simulink model "controller_dev_sg_HIL_noTP"  (R2018b)
settings: configuration reference "Physics" (kept outside this file)
model workspace (MAT data in the model file):
  m = 1000
values from neighbouring files (symbols this model uses):
  bool_activate_Vehicles : value not decoded    [controller_dev_sg.sldd]
  ModObj_ObjList_SendPort = 11004.0    [UDPPortConfig.sldd]
  ModSens_GpsSenDat_SendPort = 3002.0    [UDPPortConfig.sldd]
  sensors_freq_camera = 37.0    [controller_dev_sg.sldd]
  sensors_freq_gps = 20.0    [controller_dev_sg.sldd]
  sensors_freq_imu = 100.0    [controller_dev_sg.sldd]
  sensors_freq_lidar = 12.0    [controller_dev_sg.sldd]
  sensors_freq_radar = 20.0    [controller_dev_sg.sldd]
undefined symbols (not defined in the file or in its folder): activate_VariableFriction, C, tpa_map_Reference, tSPhysics, x0_vehiclepos_start_veh1, x0_vehiclepos_start_veh10, x0_vehiclepos_start_veh2, x0_vehiclepos_start_veh3, x0_vehiclepos_start_veh4, x0_vehiclepos_start_veh5, x0_vehiclepos_start_veh6, x0_vehiclepos_start_veh7, x0_vehiclepos_start_veh8, x0_vehiclepos_start_veh9
libraries: xpcutilitieslib x273, xpcrtudplib x215, aerolibconvert2 x48, simulink x30, etargetslib x26, speedgoatlib_IO612 x7, canmsglib x6, slrtlib x4
(part 4 of 16)

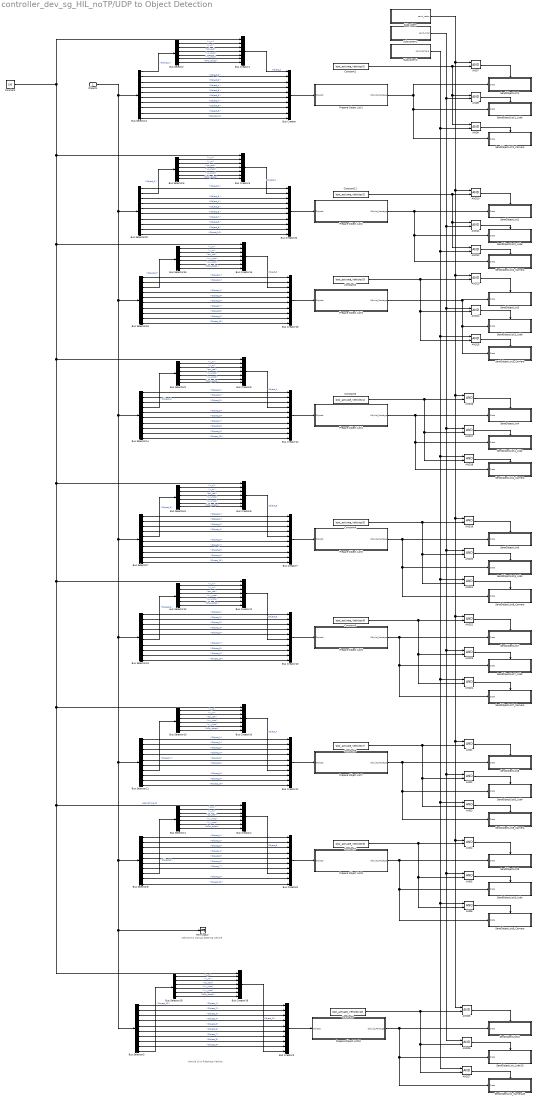
== system controller_dev_sg_HIL_noTP/UDP to Object Detection ==
  note: Vehicle 9 is Manual Steering Vehicle
  note: Vehicle 10 is Roborace Vehicle
  Objects : Inport
  AND{1..27} (27 alike) : Logic  OutDataTypeStr=boolean
  Bus Creator{,3,7..8,11,13..14,16,20} (9 alike) : BusCreator  Inputs=10
  Bus Creator{1,4..6,9..10,12,15,19} (9 alike) : BusCreator  Inputs=7
  Bus Selector{,4..6,9..10,12,15,19} (9 alike) : BusSelector  OutputSignals=x_m,y_m,psi_rad,vx_mps,vy_mps,dPsi_radps
  Bus Selector{1,3,7..8,11,13..14,16,20} (9 alike) : BusSelector  OutputSignals=Object_1,Object_2,Object_3,Object_4,Object_5,Object_6,Object_7,Object_8,Object_9,Object_10
  Constant : Constant  Value=100
  Constant1 : Constant  Value=bool_activate_Vehicles(1)  OutDataTypeStr=boolean
  Constant11 : Constant  Value=bool_activate_Vehicles(2)  OutDataTypeStr=boolean
  Constant2 : Constant  Value=bool_activate_Vehicles(3)  OutDataTypeStr=boolean
  Constant3 : Constant  Value=bool_activate_Vehicles(4)  OutDataTypeStr=boolean
  Constant4 : Constant  Value=bool_activate_Vehicles(5)  OutDataTypeStr=boolean
  Constant5 : Constant  Value=bool_activate_Vehicles(6)  OutDataTypeStr=boolean
  Constant6 : Constant  Value=bool_activate_Vehicles(7)  OutDataTypeStr=boolean
  Constant7 : Constant  Value=bool_activate_Vehicles(8)  OutDataTypeStr=boolean
  Constant8 : Constant  Value=bool_activate_Vehicles(10)  OutDataTypeStr=boolean
  Prepare Object List1 : Subsystem
  Prepare Object List10 : Subsystem
  Prepare Object List2 : Subsystem
  Prepare Object List3 : Subsystem
  Prepare Object List4 : Subsystem
  Prepare Object List5 : Subsystem
  Prepare Object List6 : Subsystem
  Prepare Object List7 : Subsystem
  Prepare Object List8 : Subsystem
  SendObjectList1 : Subsystem
  SendObjectList10 : Subsystem
  SendObjectList1_Camera : Subsystem
  SendObjectList1_Lidar : Subsystem
  SendObjectList2 : Subsystem
  SendObjectList2_Camera : Subsystem
  SendObjectList2_Lidar : Subsystem
  SendObjectList3 : Subsystem
  SendObjectList3_Camera : Subsystem
  SendObjectList3_Lidar : Subsystem
  SendObjectList4 : Subsystem
  SendObjectList4_Camera : Subsystem
  SendObjectList4_Lidar : Subsystem
  SendObjectList6 : Subsystem
  SendObjectList6_Camera : Subsystem
  SendObjectList6_Lidar : Subsystem
  SendObjectList7 : Subsystem
  SendObjectList7_Camera : Subsystem
  SendObjectList7_Lidar : Subsystem
  SendObjectList8 : Subsystem
  SendObjectList8_Camera : Subsystem
  SendObjectList8_Lidar : Subsystem
  SendObjectList9 : Subsystem
  SendObjectList9_Camera : Subsystem
  SendObjectList9_Lidar : Subsystem
  SendObjectList_Camera10 : Subsystem
  SendObjectList_Lidar10 : Subsystem
  Subsystem : Subsystem
  Subsystem1 : Subsystem
  Subsystem2 : Subsystem
  Terminator : Terminator
  wires:
  Constant1/1 -> AND7/2, AND9/1, AND8/1
  Bus Selector1/4 -> Bus Creator/4  "<Object_4>"
  Bus Selector1/3 -> Bus Creator/3  "<Object_3>"
  Bus Selector1/2 -> Bus Creator/2  "<Object_2>"
  Bus Creator/1 -> Prepare Object List1/1(Objects)
  Bus Selector1/1 -> Bus Selector/1  "<Object_1>"
  Bus Selector/6 -> Bus Creator1/7  "<dPsi_radps>"
  Bus Selector/5 -> Bus Creator1/6  "<vy_mps>"
  Bus Selector/4 -> Bus Creator1/5  "<vx_mps>"
  Bus Selector/3 -> Bus Creator1/4  "<psi_rad>"
  Bus Selector/2 -> Bus Creator1/3  "<y_m>"
  Bus Selector/1 -> Bus Creator1/2  "<x_m>"
  Bus Creator1/1 -> Bus Creator/1  "Object_1"
  Bus Selector5/3 -> Bus Creator5/4  "<psi_rad>"
  Bus Selector5/1 -> Bus Creator5/2  "<x_m>"
  Bus Selector5/2 -> Bus Creator5/3  "<y_m>"
  Bus Selector5/6 -> Bus Creator5/7  "<dPsi_radps>"
  Bus Selector5/5 -> Bus Creator5/6  "<vy_mps>"
  Bus Selector5/4 -> Bus Creator5/5  "<vx_mps>"
  Bus Selector1/5 -> Bus Creator/5  "<Object_5>"
  Bus Selector1/6 -> Bus Creator/6  "<Object_6>"
  AND7/1 -> SendObjectList1/Enable
  AND11/1 -> SendObjectList2_Lidar/Enable
  Constant11/1 -> AND10/2, AND12/1, AND11/1
  AND10/1 -> SendObjectList2/Enable
  AND12/1 -> SendObjectList2_Camera/Enable
  AND13/1 -> SendObjectList3/Enable
  AND14/1 -> SendObjectList3_Lidar/Enable
  AND15/1 -> SendObjectList3_Camera/Enable
  Constant2/1 -> AND13/2, AND14/2, AND15/2
  AND16/1 -> SendObjectList4/Enable
  AND17/1 -> SendObjectList4_Lidar/Enable
  AND18/1 -> SendObjectList4_Camera/Enable
  Constant3/1 -> AND16/2, AND17/2, AND18/2
  Constant4/1 -> AND21/2, AND20/2, AND19/2
  AND20/1 -> SendObjectList6_Lidar/Enable
  AND19/1 -> SendObjectList6/Enable
  AND21/1 -> SendObjectList6_Camera/Enable
  Constant5/1 -> AND24/2, AND23/2, AND22/2
  AND22/1 -> SendObjectList7/Enable
  AND23/1 -> SendObjectList7_Lidar/Enable
  AND24/1 -> SendObjectList7_Camera/Enable
  Prepare Object List1/1(ObjList_Package) -> SendObjectList1/1(Data), SendObjectList1_Camera/1(Data), SendObjectList1_Lidar/1(Data)
  Prepare Object List2/1(ObjList_Package) -> SendObjectList2/1(Data), SendObjectList2_Camera/1(Data), SendObjectList2_Lidar/1(Data)
  Prepare Object List3/1(ObjList_Package) -> SendObjectList3/1(Data), SendObjectList3_Camera/1(Data), SendObjectList3_Lidar/1(Data)
  Prepare Object List4/1(ObjList_Package) -> SendObjectList4/1(Data), SendObjectList4_Camera/1(Data), SendObjectList4_Lidar/1(Data)
  Prepare Object List5/1(ObjList_Package) -> SendObjectList6/1(Data), SendObjectList6_Camera/1(Data), SendObjectList6_Lidar/1(Data)
  Prepare Object List6/1(ObjList_Package) -> SendObjectList7/1(Data), SendObjectList7_Camera/1(Data), SendObjectList7_Lidar/1(Data)
  Bus Selector1/7 -> Bus Creator/7  "<Object_7>"
  Bus Selector1/8 -> Bus Creator/8  "<Object_8>"
  Bus Selector1/9 -> Bus Creator/9  "<Object_9>"
  Bus Selector1/10 -> Bus Creator/10  "<Object_10>"
  Prepare Object List8/1(ObjList_Package) -> SendObjectList9/1(Data), SendObjectList9_Camera/1(Data), SendObjectList9_Lidar/1(Data)
  Prepare Object List7/1(ObjList_Package) -> SendObjectList8/1(Data), SendObjectList8_Camera/1(Data), SendObjectList8_Lidar/1(Data)
  AND1/1 -> SendObjectList8/Enable
  AND4/1 -> SendObjectList9/Enable
  AND5/1 -> SendObjectList9_Lidar/Enable
  Constant7/1 -> AND6/2, AND5/2, AND4/2
  AND3/1 -> SendObjectList8_Camera/Enable
  Constant6/1 -> AND3/2, AND2/2, AND1/2
  AND2/1 -> SendObjectList8_Lidar/Enable
  AND6/1 -> SendObjectList9_Camera/Enable
  Prepare Object List10/1(ObjList_Package) -> SendObjectList10/1(Data), SendObjectList_Lidar10/1(Data), SendObjectList_Camera10/1(Data)
  Subsystem2/1(send_camera) -> AND27/1, AND6/1, AND3/1, AND24/1, AND21/1, AND18/1, AND15/1, AND12/2, AND9/2
  AND25/1 -> SendObjectList10/Enable
  Bus Selector19/5 -> Bus Creator19/6  "<vy_mps>"
  Bus Selector19/2 -> Bus Creator19/3  "<y_m>"
  AND27/1 -> SendObjectList_Camera10/Enable
  Bus Selector19/1 -> Bus Creator19/2  "<x_m>"
  Subsystem/1(send_radar) -> AND25/1, AND4/1, AND1/1, AND22/1, AND19/1, AND16/1, AND13/1, AND10/1, AND7/1
  Constant8/1 -> AND27/2, AND26/2, AND25/2
  Subsystem1/1(send_lidar) -> AND26/1, AND5/1, AND2/1, AND23/1, AND20/1, AND17/1, AND14/1, AND11/2, AND8/2
  Bus Selector19/4 -> Bus Creator19/5  "<vx_mps>"
  AND26/1 -> SendObjectList_Lidar10/Enable
  Bus Selector19/6 -> Bus Creator19/7  "<dPsi_radps>"
  Bus Selector19/3 -> Bus Creator19/4  "<psi_rad>"
  Bus Selector20/5 -> Bus Creator20/5  "<Object_5>"
  Bus Selector20/3 -> Bus Creator20/3  "<Object_3>"
  Bus Selector20/4 -> Bus Creator20/4  "<Object_4>"
  Bus Selector20/9 -> Bus Creator20/9  "<Object_9>"
  Bus Selector20/10 -> Bus Creator20/10  "<Object_10>"
  Bus Selector20/7 -> Bus Creator20/7  "<Object_7>"
  Bus Selector20/6 -> Bus Creator20/6  "<Object_6>"
  Bus Selector20/8 -> Bus Creator20/8  "<Object_8>"
  Bus Creator20/1 -> Prepare Object List2/1(Objects)
  Bus Selector20/2 -> Bus Selector5/1  "<Object_2>"
  Bus Creator5/1 -> Bus Creator20/2  "Object_2"
  Bus Selector20/1 -> Bus Creator20/1  "<Object_1>"
  Bus Selector3/7 -> Bus Creator3/7  "<Object_7>"
  Bus Selector3/2 -> Bus Creator3/2  "<Object_2>"
  Bus Selector3/3 -> Bus Creator3/3  "<Object_3>"
  Bus Selector3/6 -> Bus Creator3/6  "<Object_6>"
  Bus Selector3/4 -> Bus Creator3/4  "<Object_4>"
  Bus Creator3/1 -> Prepare Object List10/1(Objects)
  Bus Selector3/8 -> Bus Creator3/8  "<Object_8>"
  Bus Selector3/5 -> Bus Creator3/5  "<Object_5>"
  Bus Selector3/1 -> Bus Creator3/1  "<Object_1>"
  Bus Selector3/10 -> Bus Selector19/1  "<Object_10>"
  Bus Creator19/1 -> Bus Creator3/10  "Object_10"
  Bus Selector4/2 -> Bus Creator4/3  "<y_m>"
  Bus Selector4/5 -> Bus Creator4/6  "<vy_mps>"
  Bus Selector4/6 -> Bus Creator4/7  "<dPsi_radps>"
  Bus Selector4/3 -> Bus Creator4/4  "<psi_rad>"
  Bus Selector4/4 -> Bus Creator4/5  "<vx_mps>"
  Bus Selector8/10 -> Bus Creator8/10  "<Object_10>"
  Bus Selector8/4 -> Bus Creator8/4  "<Object_4>"
  Bus Selector8/6 -> Bus Creator8/6  "<Object_6>"
  Bus Selector8/7 -> Bus Creator8/7  "<Object_7>"
  Bus Selector4/1 -> Bus Creator4/2  "<x_m>"
  Bus Selector8/5 -> Bus Creator8/5  "<Object_5>"
  Bus Selector8/1 -> Bus Creator8/1  "<Object_1>"
  Bus Selector8/3 -> Bus Creator8/3  "<Object_3>"
  Bus Creator8/1 -> Prepare Object List8/1(Objects)
  Bus Selector8/2 -> Bus Creator8/2  "<Object_2>"
  Bus Selector8/9 -> Bus Creator8/9  "<Object_9>"
  Bus Selector8/8 -> Bus Selector4/1  "<Object_8>"
  Bus Creator4/1 -> Bus Creator8/8  "Object_8"
  Bus Selector10/2 -> Bus Creator10/3  "<y_m>"
  Bus Selector10/5 -> Bus Creator10/6  "<vy_mps>"
  Bus Selector10/6 -> Bus Creator10/7  "<dPsi_radps>"
  Bus Selector10/3 -> Bus Creator10/4  "<psi_rad>"
  Bus Selector10/4 -> Bus Creator10/5  "<vx_mps>"
  Bus Selector11/10 -> Bus Creator11/10  "<Object_10>"
  Bus Selector11/4 -> Bus Creator11/4  "<Object_4>"
  Bus Selector11/6 -> Bus Creator11/6  "<Object_6>"
  Bus Selector10/1 -> Bus Creator10/2  "<x_m>"
  Bus Selector11/5 -> Bus Creator11/5  "<Object_5>"
  Bus Selector11/8 -> Bus Creator11/8  "<Object_8>"
  Bus Selector11/1 -> Bus Creator11/1  "<Object_1>"
  Bus Selector11/3 -> Bus Creator11/3  "<Object_3>"
  Bus Creator11/1 -> Prepare Object List7/1(Objects)
  Bus Selector11/2 -> Bus Creator11/2  "<Object_2>"
  Bus Selector11/7 -> Bus Selector10/1  "<Object_7>"
  Bus Creator10/1 -> Bus Creator11/7  "Object_7"
  Bus Selector11/9 -> Bus Creator11/9  "<Object_9>"
  Bus Selector12/2 -> Bus Creator12/3  "<y_m>"
  Bus Selector12/5 -> Bus Creator12/6  "<vy_mps>"
  Bus Selector12/6 -> Bus Creator12/7  "<dPsi_radps>"
  Bus Selector12/3 -> Bus Creator12/4  "<psi_rad>"
  Bus Selector12/4 -> Bus Creator12/5  "<vx_mps>"
  Bus Selector13/10 -> Bus Creator13/10  "<Object_10>"
  Bus Selector13/4 -> Bus Creator13/4  "<Object_4>"
  Bus Selector13/7 -> Bus Creator13/7  "<Object_7>"
  Bus Selector12/1 -> Bus Creator12/2  "<x_m>"
  Bus Selector13/5 -> Bus Creator13/5  "<Object_5>"
  Bus Selector13/8 -> Bus Creator13/8  "<Object_8>"
  Bus Selector13/1 -> Bus Creator13/1  "<Object_1>"
  Bus Selector13/3 -> Bus Creator13/3  "<Object_3>"
  Bus Creator13/1 -> Prepare Object List6/1(Objects)
  Bus Selector13/2 -> Bus Creator13/2  "<Object_2>"
  Bus Selector13/6 -> Bus Selector12/1  "<Object_6>"
  Bus Creator12/1 -> Bus Creator13/6  "Object_6"
  Bus Selector13/9 -> Bus Creator13/9  "<Object_9>"
  Bus Selector6/2 -> Bus Creator6/3  "<y_m>"
  Bus Selector6/5 -> Bus Creator6/6  "<vy_mps>"
  Bus Selector6/6 -> Bus Creator6/7  "<dPsi_radps>"
  Bus Selector6/3 -> Bus Creator6/4  "<psi_rad>"
  Bus Selector6/4 -> Bus Creator6/5  "<vx_mps>"
  Bus Selector7/10 -> Bus Creator7/10  "<Object_10>"
  Bus Selector7/4 -> Bus Creator7/4  "<Object_4>"
  Bus Selector7/7 -> Bus Creator7/7  "<Object_7>"
  Bus Selector6/1 -> Bus Creator6/2  "<x_m>"
  Bus Selector7/8 -> Bus Creator7/8  "<Object_8>"
  Constant/1 -> Bus Creator1/1, Bus Creator15/1, Bus Creator9/1, Bus Creator6/1, Bus Creator12/1, Bus Creator10/1, Bus Creator4/1, Bus Creator19/1, Bus Creator5/1  "egoVehicle_ID"
  Bus Selector7/1 -> Bus Creator7/1  "<Object_1>"
  Bus Selector7/3 -> Bus Creator7/3  "<Object_3>"
  Bus Creator7/1 -> Prepare Object List5/1(Objects)
  Bus Selector7/2 -> Bus Creator7/2  "<Object_2>"
  Bus Selector9/2 -> Bus Creator9/3  "<y_m>"
  Bus Selector9/5 -> Bus Creator9/6  "<vy_mps>"
  Bus Selector9/6 -> Bus Creator9/7  "<dPsi_radps>"
  Bus Selector9/3 -> Bus Creator9/4  "<psi_rad>"
  Bus Selector9/4 -> Bus Creator9/5  "<vx_mps>"
  Bus Selector14/10 -> Bus Creator14/10  "<Object_10>"
  Bus Selector14/6 -> Bus Creator14/6  "<Object_6>"
  Bus Selector14/7 -> Bus Creator14/7  "<Object_7>"
  Bus Selector9/1 -> Bus Creator9/2  "<x_m>"
  Bus Selector14/5 -> Bus Creator14/5  "<Object_5>"
  Bus Selector14/8 -> Bus Creator14/8  "<Object_8>"
  Bus Selector14/1 -> Bus Creator14/1  "<Object_1>"
  Bus Selector14/3 -> Bus Creator14/3  "<Object_3>"
  Bus Creator14/1 -> Prepare Object List4/1(Objects)
  Bus Selector14/2 -> Bus Creator14/2  "<Object_2>"
  Bus Selector15/2 -> Bus Creator15/3  "<y_m>"
  Bus Selector15/5 -> Bus Creator15/6  "<vy_mps>"
  Bus Selector15/6 -> Bus Creator15/7  "<dPsi_radps>"
  Bus Selector15/3 -> Bus Creator15/4  "<psi_rad>"
  Bus Selector15/4 -> Bus Creator15/5  "<vx_mps>"
  Bus Selector16/10 -> Bus Creator16/10  "<Object_10>"
  Bus Selector16/4 -> Bus Creator16/4  "<Object_4>"
  Bus Selector16/6 -> Bus Creator16/6  "<Object_6>"
  Bus Selector16/7 -> Bus Creator16/7  "<Object_7>"
  Bus Selector15/1 -> Bus Creator15/2  "<x_m>"
  Bus Selector16/5 -> Bus Creator16/5  "<Object_5>"
  Bus Selector16/8 -> Bus Creator16/8  "<Object_8>"
  Bus Selector16/1 -> Bus Creator16/1  "<Object_1>"
  Objects/1 -> Bus Selector20/1, Bus Selector16/1, Bus Selector14/1, Bus Selector7/1, Bus Selector13/1, Bus Selector11/1, Bus Selector8/1, Bus Selector3/1, Terminator/1, Bus Selector1/1
  Bus Creator16/1 -> Prepare Object List3/1(Objects)
  Bus Selector16/2 -> Bus Creator16/2  "<Object_2>"
  Bus Selector16/9 -> Bus Creator16/9  "<Object_9>"
  Bus Selector16/3 -> Bus Selector15/1  "<Object_3>"
  Bus Creator15/1 -> Bus Creator16/3  "Object_3"
  Bus Selector14/4 -> Bus Selector9/1  "<Object_4>"
  Bus Creator9/1 -> Bus Creator14/4  "Object_4"
  Bus Selector14/9 -> Bus Creator14/9  "<Object_9>"
  Bus Selector7/9 -> Bus Creator7/9  "<Object_9>"
  Bus Selector7/5 -> Bus Selector6/1  "<Object_5>"
  Bus Creator6/1 -> Bus Creator7/5  "Object_5"
  Bus Selector7/6 -> Bus Creator7/6  "<Object_6>"
  AND8/1 -> SendObjectList1_Lidar/Enable
  AND9/1 -> SendObjectList1_Camera/Enable
  Bus Selector3/9 -> Bus Creator3/9  "<Object_9>"

== system controller_dev_sg_HIL_noTP/UDP to Sensors (GNSS, IMU) ==
  VehicleSensorData : Inport
  SimRealState : Inport  Port=2
  Enable : EnablePort  ShowOutputPort=on
  BESTPOS : Subsystem
  BESTUTM : Subsystem
  BESTVAL : Subsystem
  CORRIMUDATA : Subsystem
  DUALANTENNAHEADING : Subsystem
  INSPVA : Subsystem
  Logical Operator : Logic  AllPortsSameDT=off  OutDataTypeStr=boolean
  Logical Operator1 : Logic  AllPortsSameDT=off  OutDataTypeStr=boolean
  PSRDOP2 : Subsystem
  RAWIMU : Subsystem
  Subsystem : Subsystem
  Subsystem1 : Subsystem
  wires:
  Logical Operator1/1 -> CORRIMUDATA/Enable, RAWIMU/Enable
  VehicleSensorData/1 -> CORRIMUDATA/1(VehicleSensorData), BESTPOS/1(VehicleSensorData), BESTVAL/1(VehicleSensorData), DUALANTENNAHEADING/1(VehicleSensorData), RAWIMU/1(VehicleSensorData), INSPVA/1(VehicleSensorData), BESTUTM/1(VehicleSensorData)
  SimRealState/1 -> DUALANTENNAHEADING/2(SimRealState), INSPVA/2(SimRealState), BESTVAL/2(SimRealState)
  Logical Operator/1 -> DUALANTENNAHEADING/Enable, INSPVA/Enable, BESTUTM/Enable, PSRDOP2/Enable, BESTVAL/Enable, BESTPOS/Enable
  Enable/1 -> Logical Operator1/1, Logical Operator/1
  Subsystem/1(send_gps) -> Logical Operator/2
  Subsystem1/1(send_imu) -> Logical Operator1/2

== system controller_dev_sg_HIL_noTP/UDP to Sensors (GNSS, IMU)1 ==
  VehicleSensorData : Inport
  SimRealState : Inport  Port=2
  Enable : EnablePort  ShowOutputPort=on
  BESTPOS : Subsystem
  BESTUTM : Subsystem
  BESTVAL : Subsystem
  CORRIMUDATA : Subsystem
  DUALANTENNAHEADING : Subsystem
  INSPVA : Subsystem
  Logical Operator : Logic  AllPortsSameDT=off  OutDataTypeStr=boolean
  Logical Operator1 : Logic  AllPortsSameDT=off  OutDataTypeStr=boolean
  PSRDOP2 : Subsystem
  RAWIMU : Subsystem
  Subsystem : Subsystem
  Subsystem1 : Subsystem
  wires:
  Logical Operator1/1 -> RAWIMU/Enable, CORRIMUDATA/Enable
  VehicleSensorData/1 -> CORRIMUDATA/1(VehicleSensorData), BESTPOS/1(VehicleSensorData), BESTVAL/1(VehicleSensorData), DUALANTENNAHEADING/1(VehicleSensorData), RAWIMU/1(VehicleSensorData), INSPVA/1(VehicleSensorData), BESTUTM/1(VehicleSensorData)
  SimRealState/1 -> DUALANTENNAHEADING/2(SimRealState), INSPVA/2(SimRealState), BESTVAL/2(SimRealState)
  Logical Operator/1 -> BESTPOS/Enable, DUALANTENNAHEADING/Enable, INSPVA/Enable, BESTUTM/Enable, PSRDOP2/Enable, BESTVAL/Enable
  Enable/1 -> Logical Operator1/1, Logical Operator/1
  Subsystem/1(send_gps) -> Logical Operator/2
  Subsystem1/1(send_imu) -> Logical Operator1/2

== system controller_dev_sg_HIL_noTP/UDP to Sensors (GNSS, IMU)2 ==
  VehicleSensorData : Inport
  SimRealState : Inport  Port=2
  Enable : EnablePort  ShowOutputPort=on
  BESTPOS : Subsystem
  BESTUTM : Subsystem
  BESTVAL : Subsystem
  CORRIMUDATA : Subsystem
  DUALANTENNAHEADING : Subsystem
  INSPVA : Subsystem
  Logical Operator : Logic  AllPortsSameDT=off  OutDataTypeStr=boolean
  Logical Operator1 : Logic  AllPortsSameDT=off  OutDataTypeStr=boolean
  PSRDOP2 : Subsystem
  RAWIMU : Subsystem
  Subsystem : Subsystem
  Subsystem1 : Subsystem
  wires:
  Logical Operator1/1 -> RAWIMU/Enable, CORRIMUDATA/Enable
  VehicleSensorData/1 -> CORRIMUDATA/1(VehicleSensorData), BESTPOS/1(VehicleSensorData), BESTVAL/1(VehicleSensorData), DUALANTENNAHEADING/1(VehicleSensorData), RAWIMU/1(VehicleSensorData), INSPVA/1(VehicleSensorData), BESTUTM/1(VehicleSensorData)
  SimRealState/1 -> DUALANTENNAHEADING/2(SimRealState), INSPVA/2(SimRealState), BESTVAL/2(SimRealState)
  Logical Operator/1 -> BESTPOS/Enable, DUALANTENNAHEADING/Enable, INSPVA/Enable, BESTUTM/Enable, PSRDOP2/Enable, BESTVAL/Enable
  Enable/1 -> Logical Operator1/1, Logical Operator/1
  Subsystem/1(send_gps) -> Logical Operator/2
  Subsystem1/1(send_imu) -> Logical Operator1/2

== system controller_dev_sg_HIL_noTP/UDP to Sensors (GNSS, IMU)3 ==
  VehicleSensorData : Inport
  SimRealState : Inport  Port=2
  Enable : EnablePort  ShowOutputPort=on
  BESTPOS : Subsystem
  BESTUTM : Subsystem
  BESTVAL : Subsystem
  CORRIMUDATA : Subsystem
  DUALANTENNAHEADING : Subsystem
  INSPVA : Subsystem
  Logical Operator : Logic  AllPortsSameDT=off  OutDataTypeStr=boolean
  Logical Operator1 : Logic  AllPortsSameDT=off  OutDataTypeStr=boolean
  PSRDOP2 : Subsystem
  RAWIMU : Subsystem
  Subsystem : Subsystem
  Subsystem1 : Subsystem
  wires:
  Logical Operator1/1 -> RAWIMU/Enable, CORRIMUDATA/Enable
  VehicleSensorData/1 -> CORRIMUDATA/1(VehicleSensorData), BESTPOS/1(VehicleSensorData), BESTVAL/1(VehicleSensorData), DUALANTENNAHEADING/1(VehicleSensorData), RAWIMU/1(VehicleSensorData), INSPVA/1(VehicleSensorData), BESTUTM/1(VehicleSensorData)
  SimRealState/1 -> DUALANTENNAHEADING/2(SimRealState), INSPVA/2(SimRealState), BESTVAL/2(SimRealState)
  Logical Operator/1 -> BESTPOS/Enable, DUALANTENNAHEADING/Enable, INSPVA/Enable, BESTUTM/Enable, PSRDOP2/Enable, BESTVAL/Enable
  Enable/1 -> Logical Operator1/1, Logical Operator/1
  Subsystem/1(send_gps) -> Logical Operator/2
  Subsystem1/1(send_imu) -> Logical Operator1/2

== system controller_dev_sg_HIL_noTP/UDP to Sensors (GNSS, IMU)4 ==
  VehicleSensorData : Inport
  SimRealState : Inport  Port=2
  Enable : EnablePort  ShowOutputPort=on
  BESTPOS : Subsystem
  BESTUTM : Subsystem
  BESTVAL : Subsystem
  CORRIMUDATA : Subsystem
  DUALANTENNAHEADING : Subsystem
  INSPVA : Subsystem
  Logical Operator : Logic  AllPortsSameDT=off  OutDataTypeStr=boolean
  Logical Operator1 : Logic  AllPortsSameDT=off  OutDataTypeStr=boolean
  PSRDOP2 : Subsystem
  RAWIMU : Subsystem
  Subsystem : Subsystem
  Subsystem1 : Subsystem
  wires:
  Logical Operator1/1 -> RAWIMU/Enable, CORRIMUDATA/Enable
  VehicleSensorData/1 -> CORRIMUDATA/1(VehicleSensorData), BESTPOS/1(VehicleSensorData), BESTVAL/1(VehicleSensorData), DUALANTENNAHEADING/1(VehicleSensorData), RAWIMU/1(VehicleSensorData), INSPVA/1(VehicleSensorData), BESTUTM/1(VehicleSensorData)
  SimRealState/1 -> DUALANTENNAHEADING/2(SimRealState), INSPVA/2(SimRealState), BESTVAL/2(SimRealState)
  Logical Operator/1 -> BESTPOS/Enable, DUALANTENNAHEADING/Enable, INSPVA/Enable, BESTUTM/Enable, PSRDOP2/Enable, BESTVAL/Enable
  Enable/1 -> Logical Operator1/1, Logical Operator/1
  Subsystem/1(send_gps) -> Logical Operator/2
  Subsystem1/1(send_imu) -> Logical Operator1/2

== system controller_dev_sg_HIL_noTP/UDP to Sensors (GNSS, IMU)5 ==
  VehicleSensorData : Inport
  SimRealState : Inport  Port=2
  Enable : EnablePort  ShowOutputPort=on
  BESTPOS : Subsystem
  BESTUTM : Subsystem
  BESTVAL : Subsystem
  CORRIMUDATA : Subsystem
  DUALANTENNAHEADING : Subsystem
  INSPVA : Subsystem
  Logical Operator : Logic  AllPortsSameDT=off  OutDataTypeStr=boolean
  Logical Operator1 : Logic  AllPortsSameDT=off  OutDataTypeStr=boolean
  PSRDOP2 : Subsystem
  RAWIMU : Subsystem
  Subsystem : Subsystem
  Subsystem1 : Subsystem
  wires:
  Logical Operator1/1 -> RAWIMU/Enable, CORRIMUDATA/Enable
  VehicleSensorData/1 -> CORRIMUDATA/1(VehicleSensorData), BESTPOS/1(VehicleSensorData), BESTVAL/1(VehicleSensorData), DUALANTENNAHEADING/1(VehicleSensorData), RAWIMU/1(VehicleSensorData), INSPVA/1(VehicleSensorData), BESTUTM/1(VehicleSensorData)
  SimRealState/1 -> DUALANTENNAHEADING/2(SimRealState), INSPVA/2(SimRealState), BESTVAL/2(SimRealState)
  Logical Operator/1 -> BESTPOS/Enable, DUALANTENNAHEADING/Enable, INSPVA/Enable, BESTUTM/Enable, PSRDOP2/Enable, BESTVAL/Enable
  Enable/1 -> Logical Operator1/1, Logical Operator/1
  Subsystem/1(send_gps) -> Logical Operator/2
  Subsystem1/1(send_imu) -> Logical Operator1/2

== system controller_dev_sg_HIL_noTP/UDP to Sensors (GNSS, IMU)6 ==
  VehicleSensorData : Inport
  SimRealState : Inport  Port=2
  Enable : EnablePort  ShowOutputPort=on
  BESTPOS : Subsystem
  BESTUTM : Subsystem
  BESTVAL : Subsystem
  CORRIMUDATA : Subsystem
  DUALANTENNAHEADING : Subsystem
  INSPVA : Subsystem
  Logical Operator : Logic  AllPortsSameDT=off  OutDataTypeStr=boolean
  Logical Operator1 : Logic  AllPortsSameDT=off  OutDataTypeStr=boolean
  PSRDOP2 : Subsystem
  RAWIMU : Subsystem
  Subsystem : Subsystem
  Subsystem1 : Subsystem
  wires:
  Logical Operator1/1 -> RAWIMU/Enable, CORRIMUDATA/Enable
  VehicleSensorData/1 -> CORRIMUDATA/1(VehicleSensorData), BESTPOS/1(VehicleSensorData), BESTVAL/1(VehicleSensorData), DUALANTENNAHEADING/1(VehicleSensorData), RAWIMU/1(VehicleSensorData), INSPVA/1(VehicleSensorData), BESTUTM/1(VehicleSensorData)
  SimRealState/1 -> DUALANTENNAHEADING/2(SimRealState), INSPVA/2(SimRealState), BESTVAL/2(SimRealState)
  Logical Operator/1 -> BESTPOS/Enable, DUALANTENNAHEADING/Enable, INSPVA/Enable, BESTUTM/Enable, PSRDOP2/Enable, BESTVAL/Enable
  Enable/1 -> Logical Operator1/1, Logical Operator/1
  Subsystem/1(send_gps) -> Logical Operator/2
  Subsystem1/1(send_imu) -> Logical Operator1/2

== system controller_dev_sg_HIL_noTP/UDP to Sensors (GNSS, IMU)7 ==
  VehicleSensorData : Inport
  SimRealState : Inport  Port=2
  Enable : EnablePort  ShowOutputPort=on
  BESTPOS : Subsystem
  BESTUTM : Subsystem
  BESTVAL : Subsystem
  CORRIMUDATA : Subsystem
  DUALANTENNAHEADING : Subsystem
  INSPVA : Subsystem
  Logical Operator : Logic  AllPortsSameDT=off  OutDataTypeStr=boolean
  Logical Operator1 : Logic  AllPortsSameDT=off  OutDataTypeStr=boolean
  PSRDOP2 : Subsystem
  RAWIMU : Subsystem
  Subsystem : Subsystem
  Subsystem1 : Subsystem
  wires:
  Logical Operator1/1 -> RAWIMU/Enable, CORRIMUDATA/Enable
  VehicleSensorData/1 -> CORRIMUDATA/1(VehicleSensorData), BESTPOS/1(VehicleSensorData), BESTVAL/1(VehicleSensorData), DUALANTENNAHEADING/1(VehicleSensorData), RAWIMU/1(VehicleSensorData), INSPVA/1(VehicleSensorData), BESTUTM/1(VehicleSensorData)
  SimRealState/1 -> DUALANTENNAHEADING/2(SimRealState), INSPVA/2(SimRealState), BESTVAL/2(SimRealState)
  Logical Operator/1 -> BESTPOS/Enable, DUALANTENNAHEADING/Enable, INSPVA/Enable, BESTUTM/Enable, PSRDOP2/Enable, BESTVAL/Enable
  Enable/1 -> Logical Operator1/1, Logical Operator/1
  Subsystem/1(send_gps) -> Logical Operator/2
  Subsystem1/1(send_imu) -> Logical Operator1/2

== system controller_dev_sg_HIL_noTP/EnvironmentSim_Communication/Subsystem ==
  data : Inport
  "Byte Packing " : xpcutilitieslib/Byte Packing   MaskPackedDataType=uint8  MaskUnpackedDataTypes={'single'}  MaskAlignment=1
  Data Type Conversion : DataTypeConversion  OutDataTypeStr=single
  UDP Send1 : xpcrtudplib/UDP Send  ipAddressVal=10.0.0.20  localPort=12568  toAddress=10.0.0.200  toPort=50003  sampleTime=-1
      settings: SourceProductName=Simulink Real-Time  SourceProductBaseCode=XP
  Width : Width
  wires:
  data/1 -> Data Type Conversion/1
  Data Type Conversion/1 -> "Byte Packing "/1
  Width/1 -> UDP Send1/2
  "Byte Packing "/1 -> Width/1, UDP Send1/1

== system controller_dev_sg_HIL_noTP/EnvironmentSim_Communication/prepare data for sending ==
  In1 : Inport
  Add : Sum
  Add1 : Sum
  Add2 : Sum
  Bus Selector1 : BusSelector  OutputSignals=x_m,y_m,z_m,phi_rad,theta_rad,psi_rad,nWheelFL_radps,DeltaWheel_rad,nWheelFR_radps,DeltaWheel_rad,nWheelRR_radps,nWheelRL_radps,ax_mps2,ay_mps2,az_mps2,dPhi_radps,dTheta_radps,dPsi_radps,x_m,y_m,psi_rad,vx_mps,vy_mps,nWheelFL_radps,nWheelFR_radps,nWheelRR_radps,nWheelRL_radps
  Clock : Clock
  Constant{,1..5} (6 alike) : Constant  Value=0
  Constant6 : Constant
  Constant7 : Constant  Value=pi
  Constant8 : Constant  Value=pi
  Gain : Gain  Gain=0.5
  Gain1 : Gain  Gain=0.5
  Integrator{,1..3} (4 alike) : Integrator
  Math Function : Math  Operator=square  SaturateOnIntegerOverflow=on
  Math Function1 : Math  Operator=square  SaturateOnIntegerOverflow=on
  Mux : Mux  Inputs=34
  Rate Transition{,1..26} (27 alike) : RateTransition
  Sqrt : Sqrt  SaturateOnIntegerOverflow=on
  normalieAngle1 : MATLAB Function  TreatAsAtomicUnit=on
  normalieAngle2 : MATLAB Function  TreatAsAtomicUnit=on
  Out1 : Outport
  wires:
  In1/1 -> Bus Selector1/1
  Bus Selector1/12 -> Integrator3/1  "<nWheelRL_radps>"
  Gain1/1 -> Add1/1
  Gain/1 -> Add2/2
  Bus Selector1/15 -> Rate Transition14/1  "<az_mps2>"
  Rate Transition22/1 -> Mux/31
  Constant7/1 -> Gain/1
  Bus Selector1/8 -> Rate Transition9/1  "<DeltaWheel_rad>"
  Bus Selector1/22 -> Math Function1/1  "<vx_mps>"
  Rate Transition12/1 -> Mux/20
  Rate Transition13/1 -> Mux/21
  Rate Transition17/1 -> Mux/25
  Sqrt/1 -> Rate Transition21/1
  Constant5/1 -> Mux/8
  Add1/1 -> normalieAngle2/1(u)
  Math Function1/1 -> Add/1
  Constant8/1 -> Gain1/1
  Rate Transition14/1 -> Mux/22
  Math Function/1 -> Add/2
  Bus Selector1/9 -> Integrator1/1  "<nWheelFR_radps>"
  Clock/1 -> Rate Transition26/1
  normalieAngle1/1(y) -> Rate Transition20/1
  Constant4/1 -> Mux/11
  Add2/1 -> normalieAngle1/1(u)
  Constant2/1 -> Mux/16
  Bus Selector1/6 -> Add1/2  "<psi_rad>"
  Constant6/1 -> Mux/29
  Rate Transition20/1 -> Mux/28
  Bus Selector1/24 -> Rate Transition22/1  "<nWheelFL_radps>"
  Integrator2/1 -> Rate Transition10/1
  Add/1 -> Sqrt/1
  Rate Transition23/1 -> Mux/32
  Rate Transition18/1 -> Mux/26
  Rate Transition26/1 -> Mux/1
  Rate Transition25/1 -> Mux/34
  Rate Transition8/1 -> Mux/13
  Bus Selector1/23 -> Math Function/1  "<vy_mps>"
  Bus Selector1/25 -> Rate Transition23/1  "<nWheelFR_radps>"
  Rate Transition10/1 -> Mux/15
  Constant/1 -> Mux/19
  Bus Selector1/20 -> Rate Transition19/1  "<y_m>"
  Rate Transition19/1 -> Mux/27
  Constant3/1 -> Mux/14
  Bus Selector1/21 -> Add2/1  "<psi_rad>"
  Integrator1/1 -> Rate Transition7/1
  Bus Selector1/26 -> Rate Transition24/1  "<nWheelRR_radps>"
  Rate Transition9/1 -> Mux/10
  Bus Selector1/18 -> Rate Transition17/1  "<dPsi_radps>"
  Bus Selector1/19 -> Rate Transition18/1  "<x_m>"
  Bus Selector1/13 -> Rate Transition12/1  "<ax_mps2>"
  Bus Selector1/17 -> Rate Transition16/1  "<dTheta_radps>"
  Integrator3/1 -> Rate Transition11/1
  Rate Transition15/1 -> Mux/23
  Rate Transition2/1 -> Mux/7
  Rate Transition16/1 -> Mux/24
  Bus Selector1/16 -> Rate Transition15/1  "<dPhi_radps>"
  Rate Transition6/1 -> Mux/9
  Rate Transition7/1 -> Mux/12
  Bus Selector1/11 -> Integrator2/1  "<nWheelRR_radps>"
  normalieAngle2/1(y) -> Rate Transition2/1
  Bus Selector1/27 -> Rate Transition25/1  "<nWheelRL_radps>"
  Rate Transition11/1 -> Mux/18
  Bus Selector1/14 -> Rate Transition13/1  "<ay_mps2>"
  Constant1/1 -> Mux/17
  Rate Transition5/1 -> Mux/4
  Rate Transition1/1 -> Mux/3
  Bus Selector1/3 -> Rate Transition5/1  "<z_m>"
  Bus Selector1/5 -> Rate Transition3/1  "<theta_rad>"
  Bus Selector1/2 -> Rate Transition1/1  "<y_m>"
  Bus Selector1/10 -> Rate Transition8/1  "<DeltaWheel_rad>"
  Bus Selector1/7 -> Integrator/1  "<nWheelFL_radps>"
  Bus Selector1/1 -> Rate Transition/1  "<x_m>"
  Integrator/1 -> Rate Transition6/1
  Rate Transition3/1 -> Mux/6
  Bus Selector1/4 -> Rate Transition4/1  "<phi_rad>"
  Rate Transition4/1 -> Mux/5
  Rate Transition21/1 -> Mux/30
  Rate Transition24/1 -> Mux/33
  Rate Transition/1 -> Mux/2
  Mux/1 -> Out1/1

== system controller_dev_sg_HIL_noTP/EnvironmentSim_Communication/prepare data for sending1 ==
  In1 : Inport
  Add : Sum
  Add1 : Sum
  Add2 : Sum
  Bus Selector1 : BusSelector  OutputSignals=x_m,y_m,z_m,phi_rad,theta_rad,psi_rad,nWheelFL_radps,DeltaWheel_rad,nWheelFR_radps,DeltaWheel_rad,nWheelRR_radps,nWheelRL_radps,ax_mps2,ay_mps2,az_mps2,dPhi_radps,dTheta_radps,dPsi_radps,x_m,y_m,psi_rad,vx_mps,vy_mps,nWheelFL_radps,nWheelFR_radps,nWheelRR_radps,nWheelRL_radps
  Clock : Clock
  Constant{,1..5} (6 alike) : Constant  Value=0
  Constant6 : Constant
  Constant7 : Constant  Value=pi
  Constant8 : Constant  Value=pi
  Gain : Gain  Gain=0.5
  Gain1 : Gain  Gain=0.5
  Integrator{,1..3} (4 alike) : Integrator
  Math Function : Math  Operator=square  SaturateOnIntegerOverflow=on
  Math Function1 : Math  Operator=square  SaturateOnIntegerOverflow=on
  Mux : Mux  Inputs=34
  Rate Transition{,1..26} (27 alike) : RateTransition
  Sqrt : Sqrt  SaturateOnIntegerOverflow=on
  normalieAngle1 : MATLAB Function  TreatAsAtomicUnit=on
  normalieAngle2 : MATLAB Function  TreatAsAtomicUnit=on
  Out1 : Outport
  wires:
  In1/1 -> Bus Selector1/1
  Bus Selector1/12 -> Integrator3/1  "<nWheelRL_radps>"
  Gain1/1 -> Add1/1
  Gain/1 -> Add2/2
  Bus Selector1/15 -> Rate Transition14/1  "<az_mps2>"
  Rate Transition22/1 -> Mux/31
  Constant7/1 -> Gain/1
  Bus Selector1/8 -> Rate Transition9/1  "<DeltaWheel_rad>"
  Bus Selector1/22 -> Math Function1/1  "<vx_mps>"
  Rate Transition12/1 -> Mux/20
  Rate Transition13/1 -> Mux/21
  Rate Transition17/1 -> Mux/25
  Sqrt/1 -> Rate Transition21/1
  Constant5/1 -> Mux/8
  Add1/1 -> normalieAngle2/1(u)
  Math Function1/1 -> Add/1
  Constant8/1 -> Gain1/1
  Rate Transition14/1 -> Mux/22
  Math Function/1 -> Add/2
  Bus Selector1/9 -> Integrator1/1  "<nWheelFR_radps>"
  Clock/1 -> Rate Transition26/1
  normalieAngle1/1(y) -> Rate Transition20/1
  Constant4/1 -> Mux/11
  Add2/1 -> normalieAngle1/1(u)
  Constant2/1 -> Mux/16
  Bus Selector1/6 -> Add1/2  "<psi_rad>"
  Constant6/1 -> Mux/29
  Rate Transition20/1 -> Mux/28
  Bus Selector1/24 -> Rate Transition22/1  "<nWheelFL_radps>"
  Integrator2/1 -> Rate Transition10/1
  Add/1 -> Sqrt/1
  Rate Transition23/1 -> Mux/32
  Rate Transition18/1 -> Mux/26
  Rate Transition26/1 -> Mux/1
  Rate Transition25/1 -> Mux/34
  Rate Transition8/1 -> Mux/13
  Bus Selector1/23 -> Math Function/1  "<vy_mps>"
  Bus Selector1/25 -> Rate Transition23/1  "<nWheelFR_radps>"
  Rate Transition10/1 -> Mux/15
  Constant/1 -> Mux/19
  Bus Selector1/20 -> Rate Transition19/1  "<y_m>"
  Rate Transition19/1 -> Mux/27
  Constant3/1 -> Mux/14
  Bus Selector1/21 -> Add2/1  "<psi_rad>"
  Integrator1/1 -> Rate Transition7/1
  Bus Selector1/26 -> Rate Transition24/1  "<nWheelRR_radps>"
  Rate Transition9/1 -> Mux/10
  Bus Selector1/18 -> Rate Transition17/1  "<dPsi_radps>"
  Bus Selector1/19 -> Rate Transition18/1  "<x_m>"
  Bus Selector1/13 -> Rate Transition12/1  "<ax_mps2>"
  Bus Selector1/17 -> Rate Transition16/1  "<dTheta_radps>"
  Integrator3/1 -> Rate Transition11/1
  Rate Transition15/1 -> Mux/23
  Rate Transition2/1 -> Mux/7
  Rate Transition16/1 -> Mux/24
  Bus Selector1/16 -> Rate Transition15/1  "<dPhi_radps>"
  Rate Transition6/1 -> Mux/9
  Rate Transition7/1 -> Mux/12
  Bus Selector1/11 -> Integrator2/1  "<nWheelRR_radps>"
  normalieAngle2/1(y) -> Rate Transition2/1
  Bus Selector1/27 -> Rate Transition25/1  "<nWheelRL_radps>"
  Rate Transition11/1 -> Mux/18
  Bus Selector1/14 -> Rate Transition13/1  "<ay_mps2>"
  Constant1/1 -> Mux/17
  Rate Transition5/1 -> Mux/4
  Rate Transition1/1 -> Mux/3
  Bus Selector1/3 -> Rate Transition5/1  "<z_m>"
  Bus Selector1/5 -> Rate Transition3/1  "<theta_rad>"
  Bus Selector1/2 -> Rate Transition1/1  "<y_m>"
  Bus Selector1/10 -> Rate Transition8/1  "<DeltaWheel_rad>"
  Bus Selector1/7 -> Integrator/1  "<nWheelFL_radps>"
  Bus Selector1/1 -> Rate Transition/1  "<x_m>"
  Integrator/1 -> Rate Transition6/1
  Rate Transition3/1 -> Mux/6
  Bus Selector1/4 -> Rate Transition4/1  "<phi_rad>"
  Rate Transition4/1 -> Mux/5
  Rate Transition21/1 -> Mux/30
  Rate Transition24/1 -> Mux/33
  Rate Transition/1 -> Mux/2
  Mux/1 -> Out1/1

== system controller_dev_sg_HIL_noTP/EnvironmentSim_Communication/prepare data for sending2 ==
  In1 : Inport
  Add : Sum
  Add1 : Sum
  Add2 : Sum
  Bus Selector1 : BusSelector  OutputSignals=x_m,y_m,z_m,phi_rad,theta_rad,psi_rad,nWheelFL_radps,DeltaWheel_rad,nWheelFR_radps,DeltaWheel_rad,nWheelRR_radps,nWheelRL_radps,ax_mps2,ay_mps2,az_mps2,dPhi_radps,dTheta_radps,dPsi_radps,x_m,y_m,psi_rad,vx_mps,vy_mps,nWheelFL_radps,nWheelFR_radps,nWheelRR_radps,nWheelRL_radps
  Clock : Clock
  Constant{,1..5} (6 alike) : Constant  Value=0
  Constant6 : Constant
  Constant7 : Constant  Value=pi
  Constant8 : Constant  Value=pi
  Gain : Gain  Gain=0.5
  Gain1 : Gain  Gain=0.5
  Integrator{,1..3} (4 alike) : Integrator
  Math Function : Math  Operator=square  SaturateOnIntegerOverflow=on
  Math Function1 : Math  Operator=square  SaturateOnIntegerOverflow=on
  Mux : Mux  Inputs=34
  Rate Transition{,1..26} (27 alike) : RateTransition
  Sqrt : Sqrt  SaturateOnIntegerOverflow=on
  normalieAngle1 : MATLAB Function  TreatAsAtomicUnit=on
  normalieAngle2 : MATLAB Function  TreatAsAtomicUnit=on
  Out1 : Outport
  wires:
  In1/1 -> Bus Selector1/1
  Bus Selector1/12 -> Integrator3/1  "<nWheelRL_radps>"
  Gain1/1 -> Add1/1
  Gain/1 -> Add2/2
  Bus Selector1/15 -> Rate Transition14/1  "<az_mps2>"
  Rate Transition22/1 -> Mux/31
  Constant7/1 -> Gain/1
  Bus Selector1/8 -> Rate Transition9/1  "<DeltaWheel_rad>"
  Bus Selector1/22 -> Math Function1/1  "<vx_mps>"
  Rate Transition12/1 -> Mux/20
  Rate Transition13/1 -> Mux/21
  Rate Transition17/1 -> Mux/25
  Sqrt/1 -> Rate Transition21/1
  Constant5/1 -> Mux/8
  Add1/1 -> normalieAngle2/1(u)
  Math Function1/1 -> Add/1
  Constant8/1 -> Gain1/1
  Rate Transition14/1 -> Mux/22
  Math Function/1 -> Add/2
  Bus Selector1/9 -> Integrator1/1  "<nWheelFR_radps>"
  Clock/1 -> Rate Transition26/1
  normalieAngle1/1(y) -> Rate Transition20/1
  Constant4/1 -> Mux/11
  Add2/1 -> normalieAngle1/1(u)
  Constant2/1 -> Mux/16
  Bus Selector1/6 -> Add1/2  "<psi_rad>"
  Constant6/1 -> Mux/29
  Rate Transition20/1 -> Mux/28
  Bus Selector1/24 -> Rate Transition22/1  "<nWheelFL_radps>"
  Integrator2/1 -> Rate Transition10/1
  Add/1 -> Sqrt/1
  Rate Transition23/1 -> Mux/32
  Rate Transition18/1 -> Mux/26
  Rate Transition26/1 -> Mux/1
  Rate Transition25/1 -> Mux/34
  Rate Transition8/1 -> Mux/13
  Bus Selector1/23 -> Math Function/1  "<vy_mps>"
  Bus Selector1/25 -> Rate Transition23/1  "<nWheelFR_radps>"
  Rate Transition10/1 -> Mux/15
  Constant/1 -> Mux/19
  Bus Selector1/20 -> Rate Transition19/1  "<y_m>"
  Rate Transition19/1 -> Mux/27
  Constant3/1 -> Mux/14
  Bus Selector1/21 -> Add2/1  "<psi_rad>"
  Integrator1/1 -> Rate Transition7/1
  Bus Selector1/26 -> Rate Transition24/1  "<nWheelRR_radps>"
  Rate Transition9/1 -> Mux/10
  Bus Selector1/18 -> Rate Transition17/1  "<dPsi_radps>"
  Bus Selector1/19 -> Rate Transition18/1  "<x_m>"
  Bus Selector1/13 -> Rate Transition12/1  "<ax_mps2>"
  Bus Selector1/17 -> Rate Transition16/1  "<dTheta_radps>"
  Integrator3/1 -> Rate Transition11/1
  Rate Transition15/1 -> Mux/23
  Rate Transition2/1 -> Mux/7
  Rate Transition16/1 -> Mux/24
  Bus Selector1/16 -> Rate Transition15/1  "<dPhi_radps>"
  Rate Transition6/1 -> Mux/9
  Rate Transition7/1 -> Mux/12
  Bus Selector1/11 -> Integrator2/1  "<nWheelRR_radps>"
  normalieAngle2/1(y) -> Rate Transition2/1
  Bus Selector1/27 -> Rate Transition25/1  "<nWheelRL_radps>"
  Rate Transition11/1 -> Mux/18
  Bus Selector1/14 -> Rate Transition13/1  "<ay_mps2>"
  Constant1/1 -> Mux/17
  Rate Transition5/1 -> Mux/4
  Rate Transition1/1 -> Mux/3
  Bus Selector1/3 -> Rate Transition5/1  "<z_m>"
  Bus Selector1/5 -> Rate Transition3/1  "<theta_rad>"
  Bus Selector1/2 -> Rate Transition1/1  "<y_m>"
  Bus Selector1/10 -> Rate Transition8/1  "<DeltaWheel_rad>"
  Bus Selector1/7 -> Integrator/1  "<nWheelFL_radps>"
  Bus Selector1/1 -> Rate Transition/1  "<x_m>"
  Integrator/1 -> Rate Transition6/1
  Rate Transition3/1 -> Mux/6
  Bus Selector1/4 -> Rate Transition4/1  "<phi_rad>"
  Rate Transition4/1 -> Mux/5
  Rate Transition21/1 -> Mux/30
  Rate Transition24/1 -> Mux/33
  Rate Transition/1 -> Mux/2
  Mux/1 -> Out1/1

== system controller_dev_sg_HIL_noTP/EnvironmentSim_Communication/prepare data for sending3 ==
  In1 : Inport
  Add : Sum
  Add1 : Sum
  Add2 : Sum
  Bus Selector1 : BusSelector  OutputSignals=x_m,y_m,z_m,phi_rad,theta_rad,psi_rad,nWheelFL_radps,DeltaWheel_rad,nWheelFR_radps,DeltaWheel_rad,nWheelRR_radps,nWheelRL_radps,ax_mps2,ay_mps2,az_mps2,dPhi_radps,dTheta_radps,dPsi_radps,x_m,y_m,psi_rad,vx_mps,vy_mps,nWheelFL_radps,nWheelFR_radps,nWheelRR_radps,nWheelRL_radps
  Clock : Clock
  Constant{,1..5} (6 alike) : Constant  Value=0
  Constant6 : Constant
  Constant7 : Constant  Value=pi
  Constant8 : Constant  Value=pi
  Gain : Gain  Gain=0.5
  Gain1 : Gain  Gain=0.5
  Integrator{,1..3} (4 alike) : Integrator
  Math Function : Math  Operator=square  SaturateOnIntegerOverflow=on
  Math Function1 : Math  Operator=square  SaturateOnIntegerOverflow=on
  Mux : Mux  Inputs=34
  Rate Transition{,1..26} (27 alike) : RateTransition
  Sqrt : Sqrt  SaturateOnIntegerOverflow=on
  normalieAngle1 : MATLAB Function  TreatAsAtomicUnit=on
  normalieAngle2 : MATLAB Function  TreatAsAtomicUnit=on
  Out1 : Outport
  wires:
  In1/1 -> Bus Selector1/1
  Bus Selector1/12 -> Integrator3/1  "<nWheelRL_radps>"
  Gain1/1 -> Add1/1
  Gain/1 -> Add2/2
  Bus Selector1/15 -> Rate Transition14/1  "<az_mps2>"
  Rate Transition22/1 -> Mux/31
  Constant7/1 -> Gain/1
  Bus Selector1/8 -> Rate Transition9/1  "<DeltaWheel_rad>"
  Bus Selector1/22 -> Math Function1/1  "<vx_mps>"
  Rate Transition12/1 -> Mux/20
  Rate Transition13/1 -> Mux/21
  Rate Transition17/1 -> Mux/25
  Sqrt/1 -> Rate Transition21/1
  Constant5/1 -> Mux/8
  Add1/1 -> normalieAngle2/1(u)
  Math Function1/1 -> Add/1
  Constant8/1 -> Gain1/1
  Rate Transition14/1 -> Mux/22
  Math Function/1 -> Add/2
  Bus Selector1/9 -> Integrator1/1  "<nWheelFR_radps>"
  Clock/1 -> Rate Transition26/1
  normalieAngle1/1(y) -> Rate Transition20/1
  Constant4/1 -> Mux/11
  Add2/1 -> normalieAngle1/1(u)
  Constant2/1 -> Mux/16
  Bus Selector1/6 -> Add1/2  "<psi_rad>"
  Constant6/1 -> Mux/29
  Rate Transition20/1 -> Mux/28
  Bus Selector1/24 -> Rate Transition22/1  "<nWheelFL_radps>"
  Integrator2/1 -> Rate Transition10/1
  Add/1 -> Sqrt/1
  Rate Transition23/1 -> Mux/32
  Rate Transition18/1 -> Mux/26
  Rate Transition26/1 -> Mux/1
  Rate Transition25/1 -> Mux/34
  Rate Transition8/1 -> Mux/13
  Bus Selector1/23 -> Math Function/1  "<vy_mps>"
  Bus Selector1/25 -> Rate Transition23/1  "<nWheelFR_radps>"
  Rate Transition10/1 -> Mux/15
  Constant/1 -> Mux/19
  Bus Selector1/20 -> Rate Transition19/1  "<y_m>"
  Rate Transition19/1 -> Mux/27
  Constant3/1 -> Mux/14
  Bus Selector1/21 -> Add2/1  "<psi_rad>"
  Integrator1/1 -> Rate Transition7/1
  Bus Selector1/26 -> Rate Transition24/1  "<nWheelRR_radps>"
  Rate Transition9/1 -> Mux/10
  Bus Selector1/18 -> Rate Transition17/1  "<dPsi_radps>"
  Bus Selector1/19 -> Rate Transition18/1  "<x_m>"
  Bus Selector1/13 -> Rate Transition12/1  "<ax_mps2>"
  Bus Selector1/17 -> Rate Transition16/1  "<dTheta_radps>"
  Integrator3/1 -> Rate Transition11/1
  Rate Transition15/1 -> Mux/23
  Rate Transition2/1 -> Mux/7
  Rate Transition16/1 -> Mux/24
  Bus Selector1/16 -> Rate Transition15/1  "<dPhi_radps>"
  Rate Transition6/1 -> Mux/9
  Rate Transition7/1 -> Mux/12
  Bus Selector1/11 -> Integrator2/1  "<nWheelRR_radps>"
  normalieAngle2/1(y) -> Rate Transition2/1
  Bus Selector1/27 -> Rate Transition25/1  "<nWheelRL_radps>"
  Rate Transition11/1 -> Mux/18
  Bus Selector1/14 -> Rate Transition13/1  "<ay_mps2>"
  Constant1/1 -> Mux/17
  Rate Transition5/1 -> Mux/4
  Rate Transition1/1 -> Mux/3
  Bus Selector1/3 -> Rate Transition5/1  "<z_m>"
  Bus Selector1/5 -> Rate Transition3/1  "<theta_rad>"
  Bus Selector1/2 -> Rate Transition1/1  "<y_m>"
  Bus Selector1/10 -> Rate Transition8/1  "<DeltaWheel_rad>"
  Bus Selector1/7 -> Integrator/1  "<nWheelFL_radps>"
  Bus Selector1/1 -> Rate Transition/1  "<x_m>"
  Integrator/1 -> Rate Transition6/1
  Rate Transition3/1 -> Mux/6
  Bus Selector1/4 -> Rate Transition4/1  "<phi_rad>"
  Rate Transition4/1 -> Mux/5
  Rate Transition21/1 -> Mux/30
  Rate Transition24/1 -> Mux/33
  Rate Transition/1 -> Mux/2
  Mux/1 -> Out1/1

== system controller_dev_sg_HIL_noTP/EnvironmentSim_Communication/prepare data for sending4 ==
  In1 : Inport
  Add : Sum
  Add1 : Sum
  Add2 : Sum
  Bus Selector1 : BusSelector  OutputSignals=x_m,y_m,z_m,phi_rad,theta_rad,psi_rad,nWheelFL_radps,DeltaWheel_rad,nWheelFR_radps,DeltaWheel_rad,nWheelRR_radps,nWheelRL_radps,ax_mps2,ay_mps2,az_mps2,dPhi_radps,dTheta_radps,dPsi_radps,x_m,y_m,psi_rad,vx_mps,vy_mps,nWheelFL_radps,nWheelFR_radps,nWheelRR_radps,nWheelRL_radps
  Clock : Clock
  Constant{,1..5} (6 alike) : Constant  Value=0
  Constant6 : Constant
  Constant7 : Constant  Value=pi
  Constant8 : Constant  Value=pi
  Gain : Gain  Gain=0.5
  Gain1 : Gain  Gain=0.5
  Integrator{,1..3} (4 alike) : Integrator
  Math Function : Math  Operator=square  SaturateOnIntegerOverflow=on
  Math Function1 : Math  Operator=square  SaturateOnIntegerOverflow=on
  Mux : Mux  Inputs=34
  Rate Transition{,1..26} (27 alike) : RateTransition
  Sqrt : Sqrt  SaturateOnIntegerOverflow=on
  normalieAngle1 : MATLAB Function  TreatAsAtomicUnit=on
  normalieAngle2 : MATLAB Function  TreatAsAtomicUnit=on
  Out1 : Outport
  wires:
  In1/1 -> Bus Selector1/1
  Bus Selector1/12 -> Integrator3/1  "<nWheelRL_radps>"
  Gain1/1 -> Add1/1
  Gain/1 -> Add2/2
  Bus Selector1/15 -> Rate Transition14/1  "<az_mps2>"
  Rate Transition22/1 -> Mux/31
  Constant7/1 -> Gain/1
  Bus Selector1/8 -> Rate Transition9/1  "<DeltaWheel_rad>"
  Bus Selector1/22 -> Math Function1/1  "<vx_mps>"
  Rate Transition12/1 -> Mux/20
  Rate Transition13/1 -> Mux/21
  Rate Transition17/1 -> Mux/25
  Sqrt/1 -> Rate Transition21/1
  Constant5/1 -> Mux/8
  Add1/1 -> normalieAngle2/1(u)
  Math Function1/1 -> Add/1
  Constant8/1 -> Gain1/1
  Rate Transition14/1 -> Mux/22
  Math Function/1 -> Add/2
  Bus Selector1/9 -> Integrator1/1  "<nWheelFR_radps>"
  Clock/1 -> Rate Transition26/1
  normalieAngle1/1(y) -> Rate Transition20/1
  Constant4/1 -> Mux/11
  Add2/1 -> normalieAngle1/1(u)
  Constant2/1 -> Mux/16
  Bus Selector1/6 -> Add1/2  "<psi_rad>"
  Constant6/1 -> Mux/29
  Rate Transition20/1 -> Mux/28
  Bus Selector1/24 -> Rate Transition22/1  "<nWheelFL_radps>"
  Integrator2/1 -> Rate Transition10/1
  Add/1 -> Sqrt/1
  Rate Transition23/1 -> Mux/32
  Rate Transition18/1 -> Mux/26
  Rate Transition26/1 -> Mux/1
  Rate Transition25/1 -> Mux/34
  Rate Transition8/1 -> Mux/13
  Bus Selector1/23 -> Math Function/1  "<vy_mps>"
  Bus Selector1/25 -> Rate Transition23/1  "<nWheelFR_radps>"
  Rate Transition10/1 -> Mux/15
  Constant/1 -> Mux/19
  Bus Selector1/20 -> Rate Transition19/1  "<y_m>"
  Rate Transition19/1 -> Mux/27
  Constant3/1 -> Mux/14
  Bus Selector1/21 -> Add2/1  "<psi_rad>"
  Integrator1/1 -> Rate Transition7/1
  Bus Selector1/26 -> Rate Transition24/1  "<nWheelRR_radps>"
  Rate Transition9/1 -> Mux/10
  Bus Selector1/18 -> Rate Transition17/1  "<dPsi_radps>"
  Bus Selector1/19 -> Rate Transition18/1  "<x_m>"
  Bus Selector1/13 -> Rate Transition12/1  "<ax_mps2>"
  Bus Selector1/17 -> Rate Transition16/1  "<dTheta_radps>"
  Integrator3/1 -> Rate Transition11/1
  Rate Transition15/1 -> Mux/23
  Rate Transition2/1 -> Mux/7
  Rate Transition16/1 -> Mux/24
  Bus Selector1/16 -> Rate Transition15/1  "<dPhi_radps>"
  Rate Transition6/1 -> Mux/9
  Rate Transition7/1 -> Mux/12
  Bus Selector1/11 -> Integrator2/1  "<nWheelRR_radps>"
  normalieAngle2/1(y) -> Rate Transition2/1
  Bus Selector1/27 -> Rate Transition25/1  "<nWheelRL_radps>"
  Rate Transition11/1 -> Mux/18
  Bus Selector1/14 -> Rate Transition13/1  "<ay_mps2>"
  Constant1/1 -> Mux/17
  Rate Transition5/1 -> Mux/4
  Rate Transition1/1 -> Mux/3
  Bus Selector1/3 -> Rate Transition5/1  "<z_m>"
  Bus Selector1/5 -> Rate Transition3/1  "<theta_rad>"
  Bus Selector1/2 -> Rate Transition1/1  "<y_m>"
  Bus Selector1/10 -> Rate Transition8/1  "<DeltaWheel_rad>"
  Bus Selector1/7 -> Integrator/1  "<nWheelFL_radps>"
  Bus Selector1/1 -> Rate Transition/1  "<x_m>"
  Integrator/1 -> Rate Transition6/1
  Rate Transition3/1 -> Mux/6
  Bus Selector1/4 -> Rate Transition4/1  "<phi_rad>"
  Rate Transition4/1 -> Mux/5
  Rate Transition21/1 -> Mux/30
  Rate Transition24/1 -> Mux/33
  Rate Transition/1 -> Mux/2
  Mux/1 -> Out1/1
